simulink model "BasicAudio_TranslationEngine64"  (R2022b)
settings: Solver=FixedStepDiscrete  StartTime=0.0  StopTime=5  RelTol=1e-3  EnableMultiTasking=on
InitFcn:
  | % Initialize model
  | run([ ModelRootName() 'Init.m' ]);
  | 
  | % load library data
  | GainLibrary_data;
  | % Load saved values from partition process
  | CapturedConstMask.LoadMapFromFile(bdroot)
model workspace (MAT data in the model file):
  PreampVolumeTable_Idx : Simulink.Signal (value not decoded)
  Range : Simulink.Signal (value not decoded)
  Table_Idx : Simulink.Signal (value not decoded)
undefined symbols (not defined in the file or in its folder): Row
libraries: TuneVar x50, TOP x27, FeaturePath x7, CapturedConstLib x3
(part 4 of 4)

== matlab function BasicAudio_TranslationEngine64/BasicAudio/Treble/Tone/InnerLink/tone filter tune translate2 ==
  data: FilterCoeffs output; FilterFrequencyHz input; Fs input; MaskFilterType parameter
  events: trigger input FUNCTION_CALL_EVENT
function FilterCoeffs  = fcn( ...
    FilterFrequencyHz, Fs, ... % inputs
    MaskFilterType ) % parameters
%#codegen

omega = 2 * pi * FilterFrequencyHz.Value / Fs;

A = (1 - sin(omega)) / cos(omega);

if (MaskFilterType == ToneMask.TypeLowpass)
    % lowpass coeffs (e.g. bass)
    B0 = (1 - A) / 2;
    B1 = B0;
else
    % highpass coeffs (e.g. treble)
    B0 = (1 + A) / 2;
    B1 = 0 - B0;
end

FilterCoeffs = single([B0 B1 A]);

== matlab function BasicAudio_TranslationEngine64/BasicAudio/Bass/Tone/InnerLink/tone filter tune translate3 ==
  data: maxOut output; maxIn input
  events: trigger input FUNCTION_CALL_EVENT
function maxOut  = fcn( ...
    maxIn) ... % inputs % parameters
%#codegen

% Just make sure the maximum is a positive dB value
maxOut = single(abs(maxIn.Value));

== matlab function BasicAudio_TranslationEngine64/BasicAudio/Bass/Tone/InnerLink/tone filter tune translate4 ==
  data: maxOut output; maxIn input
  events: trigger input FUNCTION_CALL_EVENT
function maxOut  = fcn( ...
    maxIn) ... % inputs % parameters
%#codegen

% Just make sure the maximum is a positive dB value
maxOut = single(abs(maxIn.Value));

== matlab function BasicAudio_TranslationEngine64/BasicAudio/Treble/Tone/InnerLink/tone filter tune translate3 ==
  data: maxOut output; maxIn input
  events: trigger input FUNCTION_CALL_EVENT
function maxOut  = fcn( ...
    maxIn) ... % inputs % parameters
%#codegen

% Just make sure the maximum is a positive dB value
maxOut = single(abs(maxIn.Value));
